simulink model "truck_fra_oven"  (R2024a)
settings: Solver=VariableStepAuto  StartTime=0.0  StopTime=40  MaxStep=0.01  RelTol=1e-3
libraries: slpidlib x2
settings Model: Creator=hansae  LastModifiedBy=filip
settings SolverCC: AlgebraicLoopSolver=TrustRegion
settings SFSimCC: CustomCodeUndefinedFunction=UseInterfaceOnly
settings RTWCC: GPUComputeCapability=3.5

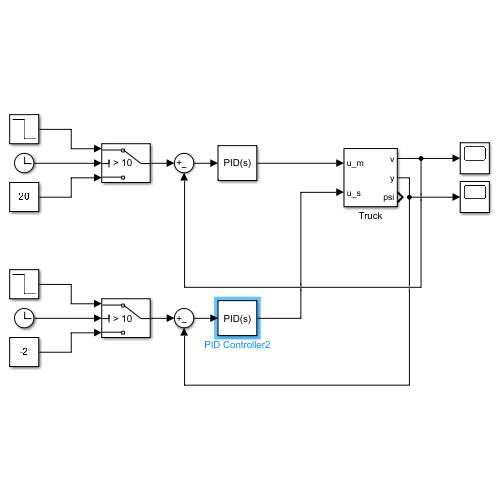
[thumbnail: Simulink's stored preview of the top-level diagram]
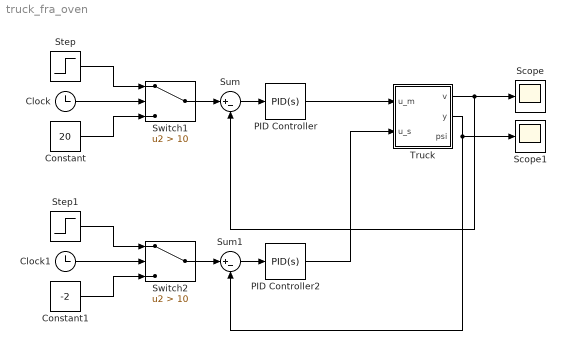
== system truck_fra_oven ==
  Clock : Clock
  Clock1 : Clock
  Constant : Constant  Value=20
  Constant1 : Constant  Value=-2
  PID Controller : slpidlib/PID Controller  Controller=PID  Form=Parallel  TimeDomain=Continuous-time  UseExternalTs=off  SampleTime=-1  IntegratorMethod=Forward Euler  FilterMethod=Forward Euler  ControllerParametersSource=internal  P=8000  I=50  UseKiTs=off  D=7500  UseExternalDerivativeSource=off  N=100  UseFilter=on  TunerSelectOption=Transfer Function Based (PID Tuner App)  InitialConditionSource=internal  InitialConditionForIntegrator=0  InitialConditionForFilter=0  DifferentiatorICPrevScaledInput=0  ExternalReset=none  TrackingMode=off  Kt=1  LimitOutput=off  SatLimitsSource=internal  UpperSaturationLimit=inf  LowerSaturationLimit=-inf  LinearizeAsGain=on  AntiWindupMode=none  Kb=1  LimitIntegrator=off  UpperIntegratorSaturationLimit=inf  LowerIntegratorSaturationLimit=-inf  POutMin=[]  POutMax=[]  IOutMin=[]  IOutMax=[]  DOutMin=[]  DOutMax=[]  NOutMin=[]  NOutMax=[]  SumOutMin=[]  SumOutMax=[]  SaturationOutMin=[]  SaturationOutMax=[]  PParamMin=[]  PParamMax=[]  IParamMin=[]  IParamMax=[]  DParamMin=[]  DParamMax=[]  NParamMin=[]  NParamMax=[]  KbParamMin=[]  KbParamMax=[]  KtParamMin=[]  KtParamMax=[]  KbOutMin=[]  KbOutMax=[]  KtOutMin=[]  KtOutMax=[]  IntegratorOutMin=[]  IntegratorOutMax=[]  FilterOutMin=[]  FilterOutMax=[]  SumI1OutMin=[]  SumI1OutMax=[]  SumI2OutMin=[]  SumI2OutMax=[]  SumI3OutMin=[]  SumI3OutMax=[]  SumI4OutMin=[]  SumI4OutMax=[]  SumDOutMin=[]  SumDOutMax=[]  DifferentiatorOutMin=[]  DifferentiatorOutMax=[]  FilterDiffOutCoefMin=[]  FilterDiffOutCoefMax=[]  ReciprocalOutMin=[]  ReciprocalOutMax=[]  SumDenOutMin=[]  SumDenOutMax=[]  SumNumOutMin=[]  SumNumOutMax=[]  DivideOutMin=[]  DivideOutMax=[]  UdiffTsProdOutMin=[]  UdiffTsProdOutMax=[]  NTsProdOutMin=[]  NTsProdOutMax=[]  UintegralTsProdOutMin=[]  UintegralTsProdOutMax=[]  UngainTsProdOutMin=[]  UngainTsProdOutMax=[]  ClampingZeroOutDataTypeStr=Inherit: Inherit via back propagation  ClampingZeroOutMin=[]  ClampingZeroOutMax=[]  FilterDenConstantOutDataTypeStr=Inherit: Inherit via back propagation  FilterDenConstantOutMin=[]  FilterDenConstantOutMax=[]  PCopyOutDataTypeStr=Inherit: Inherit via back propagation  PCopyOutMin=[]  PCopyOutMax=[]  NCopyOutDataTypeStr=Inherit: Inherit via back propagation  NCopyOutMin=[]  NCopyOutMax=[]  IntegratorContinuousStateAttributes=''  IntegratorStateMustResolveToSignalObject=off  IntegratorRTWStateStorageClass=Auto  FilterContinuousStateAttributes=''  FilterStateMustResolveToSignalObject=off  FilterRTWStateStorageClass=Auto  ParallelPVariant=InternalParameters  IdealPVariant=Disabled  IVariant=InternalParameters  DVariant=InternalParameters  IntegratorVariant=Continuous  SatVariant=Disabled  AWVariant=Passthrough  PCopyVariant=Disabled  TRVariant=Disabled  FdbkBlocksVariant=Forward  IdealPFdbkVariant=Disabled  SatFdbkVariant=Disabled  DerivativeFilterVariant=ContFilter  NVariant=InternalParameters  NCopyVariant=Disabled  FilterICVariant=InternalICsFilter  IntegratorICVariant=InternalICs  ExternalResetVariant=Disabled  TRSumVariant=Passthrough  SumFdbkVariant=Disabled  SumVariant=Sum_PID  TsampFilterVariant=InternalTs  TsampNgainVariant=Passthrough  TsampIntegralVariant=Disabled_SignalSpec  ExternalSaturationOutDataTypeStr=Inherit: Same as second input  DerivativeSourceVariant=ErrorSignal
  PID Controller2 : slpidlib/PID Controller  Controller=PID  Form=Parallel  TimeDomain=Continuous-time  UseExternalTs=off  SampleTime=-1  IntegratorMethod=Forward Euler  FilterMethod=Forward Euler  ControllerParametersSource=internal  P=0.0464198158186668  I=0.0217313338533882  UseKiTs=off  D=0.0243480245404174  UseExternalDerivativeSource=off  N=54.5397025421619  UseFilter=on  TunerSelectOption=Frequency Response Based  InitialConditionSource=internal  InitialConditionForIntegrator=0  InitialConditionForFilter=0  DifferentiatorICPrevScaledInput=0  ExternalReset=none  TrackingMode=off  Kt=1  LimitOutput=off  SatLimitsSource=internal  UpperSaturationLimit=inf  LowerSaturationLimit=-inf  LinearizeAsGain=on  AntiWindupMode=none  Kb=1  LimitIntegrator=off  UpperIntegratorSaturationLimit=inf  LowerIntegratorSaturationLimit=-inf  POutMin=[]  POutMax=[]  IOutMin=[]  IOutMax=[]  DOutMin=[]  DOutMax=[]  NOutMin=[]  NOutMax=[]  SumOutMin=[]  SumOutMax=[]  SaturationOutMin=[]  SaturationOutMax=[]  PParamMin=[]  PParamMax=[]  IParamMin=[]  IParamMax=[]  DParamMin=[]  DParamMax=[]  NParamMin=[]  NParamMax=[]  KbParamMin=[]  KbParamMax=[]  KtParamMin=[]  KtParamMax=[]  KbOutMin=[]  KbOutMax=[]  KtOutMin=[]  KtOutMax=[]  IntegratorOutMin=[]  IntegratorOutMax=[]  FilterOutMin=[]  FilterOutMax=[]  SumI1OutMin=[]  SumI1OutMax=[]  SumI2OutMin=[]  SumI2OutMax=[]  SumI3OutMin=[]  SumI3OutMax=[]  SumI4OutMin=[]  SumI4OutMax=[]  SumDOutMin=[]  SumDOutMax=[]  DifferentiatorOutMin=[]  DifferentiatorOutMax=[]  FilterDiffOutCoefMin=[]  FilterDiffOutCoefMax=[]  ReciprocalOutMin=[]  ReciprocalOutMax=[]  SumDenOutMin=[]  SumDenOutMax=[]  SumNumOutMin=[]  SumNumOutMax=[]  DivideOutMin=[]  DivideOutMax=[]  UdiffTsProdOutMin=[]  UdiffTsProdOutMax=[]  NTsProdOutMin=[]  NTsProdOutMax=[]  UintegralTsProdOutMin=[]  UintegralTsProdOutMax=[]  UngainTsProdOutMin=[]  UngainTsProdOutMax=[]  ClampingZeroOutDataTypeStr=Inherit: Inherit via back propagation  ClampingZeroOutMin=[]  ClampingZeroOutMax=[]  FilterDenConstantOutDataTypeStr=Inherit: Inherit via back propagation  FilterDenConstantOutMin=[]  FilterDenConstantOutMax=[]  PCopyOutDataTypeStr=Inherit: Inherit via back propagation  PCopyOutMin=[]  PCopyOutMax=[]  NCopyOutDataTypeStr=Inherit: Inherit via back propagation  NCopyOutMin=[]  NCopyOutMax=[]  IntegratorContinuousStateAttributes=''  IntegratorStateMustResolveToSignalObject=off  IntegratorRTWStateStorageClass=Auto  FilterContinuousStateAttributes=''  FilterStateMustResolveToSignalObject=off  FilterRTWStateStorageClass=Auto  ParallelPVariant=InternalParameters  IdealPVariant=Disabled  IVariant=InternalParameters  DVariant=InternalParameters  IntegratorVariant=Continuous  SatVariant=Disabled  AWVariant=Passthrough  PCopyVariant=Disabled  TRVariant=Disabled  FdbkBlocksVariant=Forward  IdealPFdbkVariant=Disabled  SatFdbkVariant=Disabled  DerivativeFilterVariant=ContFilter  NVariant=InternalParameters  NCopyVariant=Disabled  FilterICVariant=InternalICsFilter  IntegratorICVariant=InternalICs  ExternalResetVariant=Disabled  TRSumVariant=Passthrough  SumFdbkVariant=Disabled  SumVariant=Sum_PID  TsampFilterVariant=InternalTs  TsampNgainVariant=Passthrough  TsampIntegralVariant=Disabled_SignalSpec  ExternalSaturationOutDataTypeStr=Inherit: Same as second input  DerivativeSourceVariant=ErrorSignal
  Scope : Scope
  Scope1 : Scope
  Step : Step  Time=20  Before=30  After=20  SampleTime=0
  Step1 : Step  Time=20  Before=2  After=-2  SampleTime=0
  Sum : Sum  Inputs=|+-
  Sum1 : Sum  Inputs=|+-
  Switch1 : Switch  Criteria=u2 > Threshold  Threshold=10  SaturateOnIntegerOverflow=off  InputSameDT=off
  Switch2 : Switch  Criteria=u2 > Threshold  Threshold=10  SaturateOnIntegerOverflow=off  InputSameDT=off
  Truck : Subsystem
  wires:
  Clock/1 -> Switch1/2
  Truck/1(v) -> Scope/1, Sum/2
  Sum/1 -> PID Controller/1
  Sum1/1 -> PID Controller2/1
  Switch2/1 -> Sum1/1
  Clock1/1 -> Switch2/2
  Truck/2(y) -> Scope1/1, Sum1/2
  PID Controller2/1 -> Truck/2(u_s)
  Constant/1 -> Switch1/3
  Step/1 -> Switch1/1
  Constant1/1 -> Switch2/3
  Step1/1 -> Switch2/1
  PID Controller/1 -> Truck/1(u_m)
  Switch1/1 -> Sum/1

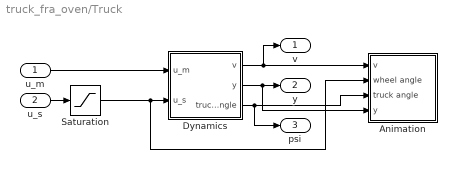
== system truck_fra_oven/Truck ==
  u_m : Inport
  u_s : Inport  Port=2
  Animation : Subsystem
  Dynamics : Subsystem  ClipboardFcn=parameters_truck.m
  Saturation : Saturate  UpperLimit=pi/4  LowerLimit=-pi/4
  v : Outport
  y : Outport  Port=2
  psi : Outport  Port=3
  wires:
  Dynamics/2(y) -> y/1, Animation/4(y)
  u_s/1 -> Saturation/1
  u_m/1 -> Dynamics/1(u_m)
  Dynamics/3(truck angle) -> psi/1, Animation/3(truck angle)
  Saturation/1 -> Animation/2(wheel angle), Dynamics/2(u_s)
  Dynamics/1(v) -> v/1, Animation/1(v)

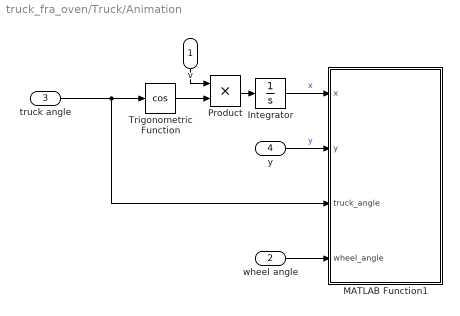
== system truck_fra_oven/Truck/Animation ==
  v : Inport
  wheel angle : Inport  Port=2
  truck angle : Inport  Port=3
  y : Inport  Port=4
  Integrator : Integrator
  MATLAB Function1 : MATLAB Function  TreatAsAtomicUnit=on  SystemSampleTime=1/30
  Product : Product
  Trigonometric Function : Trigonometry  Operator=cos
  wires:
  Product/1 -> Integrator/1
  Trigonometric Function/1 -> Product/2
  v/1 -> Product/1
  y/1 -> MATLAB Function1/2(y)  "y"
  Integrator/1 -> MATLAB Function1/1(x)  "x"
  truck angle/1 -> MATLAB Function1/3(truck_angle), Trigonometric Function/1
  wheel angle/1 -> MATLAB Function1/4(wheel_angle)

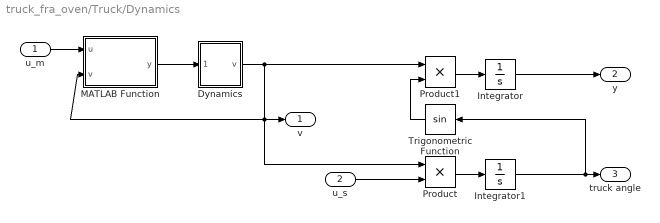
== system truck_fra_oven/Truck/Dynamics ==
  u_m : Inport
  u_s : Inport  Port=2
  Dynamics : Subsystem  ClipboardFcn=parameters_truck.m
  Integrator : Integrator  InitialCondition=-2
  Integrator1 : Integrator
  MATLAB Function : MATLAB Function  TreatAsAtomicUnit=on
  Product : Product
  Product1 : Product
  Trigonometric Function : Trigonometry
  v : Outport
  y : Outport  Port=2
  truck angle : Outport  Port=3
  wires:
  Integrator/1 -> y/1
  Product/1 -> Integrator1/1
  Product1/1 -> Integrator/1
  Trigonometric Function/1 -> Product1/2
  u_s/1 -> Product/2
  Integrator1/1 -> truck angle/1, Trigonometric Function/1
  MATLAB Function/1(y) -> Dynamics/1(u_m)
  u_m/1 -> MATLAB Function/1(u)
  Dynamics/1(v) -> Product/1, MATLAB Function/2(v), v/1, Product1/1

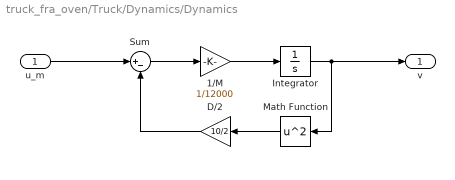
== system truck_fra_oven/Truck/Dynamics/Dynamics ==
  u_m : Inport
  1/M : Gain  Gain=1/12000
  D/2 : Gain  Gain=10/2
  Integrator : Integrator
  Math Function : Math  Operator=square  SignedPower=on
  Sum : Sum  Inputs=|+-
  v : Outport
  wires:
  Integrator/1 -> v/1, Math Function/1
  Sum/1 -> 1/M/1
  u_m/1 -> Sum/1
  1/M/1 -> Integrator/1
  D/2/1 -> Sum/2
  Math Function/1 -> D/2/1

== matlab function truck_fra_oven/Truck/Dynamics/MATLAB Function ==
  data: u input; y output; v input
function y = saturation(u,v)
    Pmax = 400000;
    epsilon = 0.1;
    
    sat = Pmax/sqrt(v^2+epsilon);
    y = max(min(u,sat),-sat);

== matlab function truck_fra_oven/Truck/Animation/MATLAB Function1 ==
  settings: updateMethod=DISCRETE
  data: x input; y input; truck_angle input; wheel_angle input
function plot_truck(x,y,truck_angle,wheel_angle)
    % Parameters
    l = 8;
    persistent Truck;

    % Plotting Truck
    if isempty(Truck)
        Truck = initialize_plot();
    else
        update_truck_position(Truck,x,y,truck_angle,wheel_angle);
    end    

    drawnow;

    % Functions
    function Truck = initialize_plot()
        % Create figure
        figure('position',[100,100,1500,500]);
        clf; grid on; hold on; daspect([1,1,1]);
        xlim([-20, 50])
        ylim([-10, 10])
    
        % Road
        plot([-5000,5000],[-4,-4],'k','linewidth',3);
        plot([-5000,5000],[4,4],'k','linewidth',3);
        plot([-5000,5000],[0,0],'y','linewidth',3);

        % Truck
        Truck               = hgtransform('parent',gca);
        Left_front_wheel    = hgtransform('parent',Truck);
        Right_front_wheel   = hgtransform('parent',Truck);

        % Back wheels
        rectangle('Position',[l/6,-l/100,l/8,l/40],'parent',Truck,'edgecolor','k','linewidth',2,'FaceColor','w')
        rectangle('Position',[l/6,l-2*l/3-(l/40-l/100),l/8,l/40],'parent',Truck,'edgecolor','k','linewidth',2,'FaceColor','w')
        % Front wheel
        rectangle('Position',[2*l/3+l/20,-l/100,l/8,l/40],'parent',Right_front_wheel,'edgecolor','k','linewidth',2,'FaceColor','w')
        rectangle('Position',[2*l/3+l/20,l-2*l/3-(l/40-l/100),l/8,l/40],'parent',Left_front_wheel,'edgecolor','k','linewidth',2,'FaceColor','w')
        % Back
        rectangle('Position',[0,0,11*l/18,l-2*l/3],'parent',Truck,'edgecolor','k','linewidth',2,'FaceColor','w')
        % Front
        rectangle('Position',[2*l/3,0,l-2*l/3,l-2*l/3],'parent',Truck,'edgecolor','k','linewidth',2,'FaceColor','w')
        % Connection
        rectangle('Position',[11*l/18,3*l/8-l/3,2*l/3-11*l/18,l-3*l/4],'parent',Truck,'edgecolor','k','linewidth',2,'FaceColor','w')
        % Window
        rectangle('Position',[7*l/8,0,l/8,l-2*l/3],'parent',Truck,'edgecolor','k','linewidth',2,'FaceColor','w')
        
    end
    
    function update_truck_position(Truck,x,y,truck_angle,wheel_angle)
        if ishandle(Truck)
            set(Truck, 'Matrix', makehgtform('translate', [x, y, 0], 'zrotate', truck_angle, 'translate', [-l/6-l/16, -l/2+l/3, 0]));
            
            children = get(Truck, 'Children');
            set(children(8), 'Matrix', makehgtform('translate', -[-(2*l/3+l/20)-l/16, -(l-2*l/3-(l/40-l/100))-l/80, 0], 'zrotate', -wheel_angle, 'translate', [-(2*l/3+l/20)-l/16, -(l-2*l/3-(l/40-l/100))-l/80, 0]));
            set(children(7), 'Matrix', makehgtform('translate', -[-(2*l/3+l/20)-l/16, l/100-l/80, 0], 'zrotate', -wheel_angle, 'translate', [-(2*l/3+l/20)-l/16, l/100-l/80, 0]));
    
            xlim([-20, 50] + x)
            ylim([-10, 10] + y)
        end
    end
end
